simulink model "DAtosInOut_PRBS"  (R2016a)
settings: Solver=ode5  StartTime=0.0  StopTime=t_ejec_anadido  RelTol=1e-3
values from neighbouring files (symbols this model uses):
  D = 1    [Genera_PRBS.m]
  ts = 0.05    [Disena_PRBS.m]    (also in RespuestaStep.m = T)
undefined symbols (not defined in the file or in its folder): sigbuilder_block
libraries: xpcnilib x3, slrtlib x3, simulink x1
Description:
  | Real-Time Controller
  | 
  | This demonstration shows how to build a simple closed-loop real-time controller using
  | Real-Time Windows Target. The output of the controlled plant is connected
  | to the analog input of your data acquisition board. This signal is subtracted from
  | the set point value generated by the signal generator and processed by a PID controller.
  | The output of the controller drives the input of the plant using the analog output
  | of your data acquisition board.
  | 
  | This model is a simplified version of the controller used for the CE152 Magnetic Levitation Model.
  | 
  | How to run this demo:
  | 
  |   1. Open the Analog Input and Analog Output blocks and select your data acquisition board.
  |       If there's no board installed, install it using the Install new board button.
  |   2. Build the model using Tools -> Real-Time Workshop -> Build Model.
  |   3. Connect to the real-time code using Simulation -> Connect to target.
  |   4. Start the real-time execution using Simulation -> Start real-time code.
  | 
  | Note:
  | To run this demo, you must have a data acquisition board plugged into your computer.
settings Model: SimulationMode=external  ExtModeTrigDuration=100000  Creator=Houska  LastModifiedBy=Ainhoa
settings SolverCC: EnableConcurrentExecution=on  AutoInsertRateTranBlk=on
settings DataIOCC: LimitDataPoints=on  MaxDataPoints=P  SaveFormat=Array  SignalLoggingSaveFormat=ModelDataLogs  SignalLoggingName=logsOut
settings OptimizationCC: BlockReduction=off  OptimizeBlockIOStorage=off  BufferReuse=off  GlobalBufferReuse=off  ExpressionFolding=off  ExpressionDepthLimit=2147483647  LocalBlockOutputs=off  InitFltsAndDblsToZero=on  EfficientMapNaN2IntZero=off
settings DebuggingCC: UnderspecifiedInitializationDetection=Classic  MergeDetectMultiDrivingBlocksExec=none  SignalResolutionControl=TryResolveAllWithWarning  FcnCallInpInsideContextMsg=UseLocalSettings  StateNameClashWarn=warning
settings HardwareCC: ProdBitPerPointer=32  ProdLargestAtomicFloat=None  ProdWordSize=32  ProdLongLongMode=on  ProdHWDeviceType=Generic->32-bit x86 compatible
settings ModelReferenceCC: PropagateSignalLabelsOutOfModel=off
settings RTWCC: SystemTargetFile=slrt.tlc  TemplateMakefile=slrt_default_tmf  Description=Simulink Real-Time  RTWCompilerOptimization=on
settings ConfigComp: CovModelRefEnable=Off

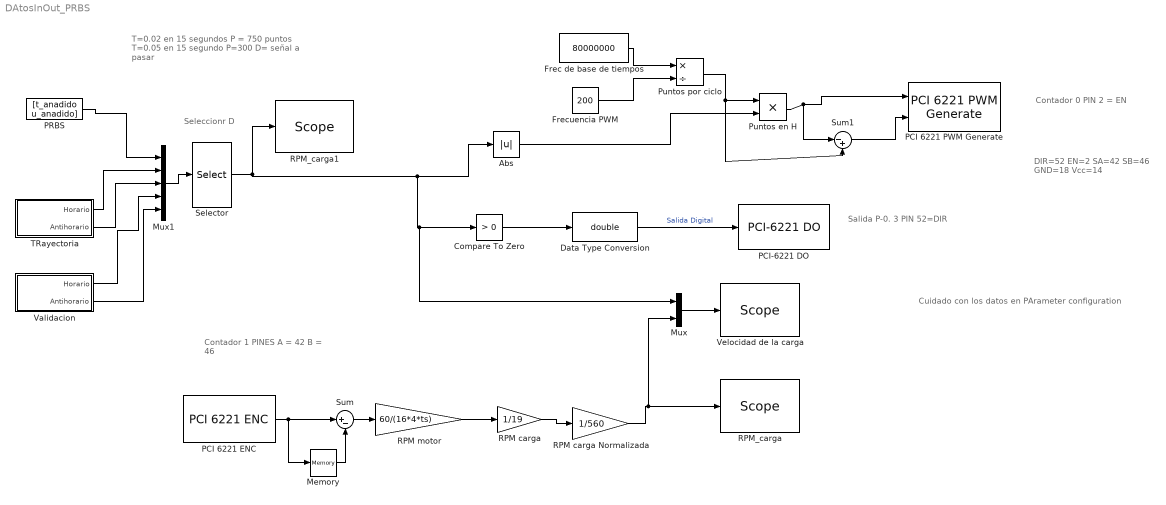
== system DAtosInOut_PRBS ==
  note: Seleccionr D
  note: T=0.02 en 15 segundos P = 750 puntos
      | T=0.05 en 15 segundo P=300
      | D= señal a pasar
  note: Cuidado con los datos en PArameter configuration
  note: DIR=52
      | EN=2
      | SA=42
      | SB=46
      | GND=18
      | Vcc=14
  note: Contador 1
      | PINES
      |  A = 42
      | B = 46
  note: Salida P-0. 3
      | PIN 52=DIR
  note: Contador 0
      | PIN 2 = EN
  Abs : Abs
  Compare To Zero : simulink/Logic and Bit Operations/Compare To Zero  relop=>  OutDataTypeStr=uint8
  Data Type Conversion : DataTypeConversion  OutDataTypeStr=double
  Frec de base de tiempos : Constant  Value=80000000
  Frecuencia PWM : Constant  Value=200
  Memory : Memory
  Mux : Mux  Inputs=2
  Mux1 : Mux  Inputs=5
  "PCI 6221 ENC " : xpcnilib/Incremental Encoder/PCI 6221 ENC   channel=1  countMode=Quadrature Mode x4  initCount=0  reload=off  indexPhase=A low B low  filter=None  sampleTime=ts  slot=-1
  "PCI 6221 PWM Generate " : xpcnilib/Counter/M Series/PCI 6221 PWM Generate   channel=0  initHigh=0  initLow=0  arm=off  disarmlevel=Disarm to LOW  stoplevel=Stop to LOW  sampletime=-1  slot=-1
  PCI-6221 DO : xpcnilib/Digital Output/M Series/PCI-6221 DO  channel=[1]  reset=[1]  initValue=[0]  sampletime=ts  slot=-1
  PRBS : FromWorkspace  VariableName=[t_anadido u_anadido]
  Puntos en H : Product  RndMeth=Zero
  Puntos por ciclo : Product  Inputs=*/
  RPM carga : Gain  Gain=1/19
  RPM carga Normalizada : Gain  Gain=1/560
  RPM motor : Gain  Gain=60/(16*4*ts)
  RPM_carga : slrtlib/Displays and Logging/Scope   scopeno=1  scopetype=File  autostart=on  viewmode=Graphical redraw  formatstr='%15.6f'  grid=on  ylimits=[0,0]  nosamples=P_anadido  noprepostsamples=0  interleave=1  triggermode=FreeRun  triggersignal=1  trigsignalfromport=off  triggerlevel=0.0  triggerslope=Either  triggerscope=1  triggersample=0  filename=salida.dat  mode=Lazy  writesize=512  autorestart=off  dynamicfilemode=off  maxwritefilesize=512*1024^2
  RPM_carga1 : slrtlib/Displays and Logging/Scope   scopeno=2  scopetype=File  autostart=on  viewmode=Graphical redraw  formatstr='%15.6f'  grid=on  ylimits=[0,0]  nosamples=P_anadido  noprepostsamples=0  interleave=1  triggermode=FreeRun  triggersignal=1  trigsignalfromport=off  triggerlevel=0.0  triggerslope=Either  triggerscope=1  triggersample=0  filename=entrada.dat  mode=Lazy  writesize=512  autorestart=off  dynamicfilemode=off  maxwritefilesize=512*1024^2
  Selector : Selector  InputPortWidth=5  IndexOptions=Index vector (dialog)  Indices=[D]  OutputSizes=1
  Sum : Sum  Inputs=|+-
  Sum1 : Sum  Inputs=|-+
  TRayectoria : Subsystem  Tag=STV Subsys  LoadFcn=sigbuilder_block('load');  StartFcn=sigbuilder_block('start');  StopFcn=sigbuilder_block('stop');  ClipboardFcn=sigbuilder_block('clipboard');  mask(Sigbuilder block){}
      mask help: Simulink:masks:SigbuilderBlock_MD
      mask init:
      | if ~strcmp(get_param(bdroot(gcbh),'SimulationStatus'),'stopped') tuvar = sigbuilder_block('maskInit'); end
      settings: CopyFcn=sigbuilder_block('copy');  DeleteFcn=sigbuilder_block('delete');  ModelCloseFcn=sigbuilder_block('modelClose');  PreSaveFcn=sigbuilder_block('preSave');  PauseFcn=sigbuilder_block('pause');  ContinueFcn=sigbuilder_block('continue');  NameChangeFcn=sigbuilder_block('namechange');  OpenFcn=sigbuilder_block('open',[6 6 1188 718.5 ]);  CloseFcn=sigbuilder_block('close');
      mask Display: plot(0, 0, 100, 100,[2, 2, 32, 32, 2], [68, 8, 8, 68, 68],[32, 2], [38, 38], [32, 19, 2],[53, 60, 44], [32, 17, 17, 2],[16, 16, 31, 31]);txt = getActiveGroup(gcbh);text(2, 100, txt,'verticalAlignment', 'top');
  Validacion : Subsystem  Tag=STV Subsys  LoadFcn=sigbuilder_block('load');  StartFcn=sigbuilder_block('start');  StopFcn=sigbuilder_block('stop');  ClipboardFcn=sigbuilder_block('clipboard');  mask(Sigbuilder block){}
      mask help: Simulink:masks:SigbuilderBlock_MD
      mask init:
      | if ~strcmp(get_param(bdroot(gcbh),'SimulationStatus'),'stopped') tuvar = sigbuilder_block('maskInit'); end
      settings: CopyFcn=sigbuilder_block('copy');  DeleteFcn=sigbuilder_block('delete');  ModelCloseFcn=sigbuilder_block('modelClose');  PreSaveFcn=sigbuilder_block('preSave');  PauseFcn=sigbuilder_block('pause');  ContinueFcn=sigbuilder_block('continue');  NameChangeFcn=sigbuilder_block('namechange');  OpenFcn=sigbuilder_block('open',[43.5 -15.75 1188 714 ]);  CloseFcn=sigbuilder_block('close');
      mask Display: plot(0, 0, 100, 100,[2, 2, 32, 32, 2], [68, 8, 8, 68, 68],[32, 2], [38, 38], [32, 19, 2],[53, 60, 44], [32, 17, 17, 2],[16, 16, 31, 31]);txt = getActiveGroup(gcbh);text(2, 100, txt,'verticalAlignment', 'top');
  Velocidad de la carga : slrtlib/Displays and Logging/Scope   scopeno=3  scopetype=Host  autostart=on  viewmode=Graphical redraw  formatstr='%15.6f'  grid=on  ylimits=[0,0]  nosamples=P_anadido  noprepostsamples=1  interleave=1  triggermode=FreeRun  triggersignal=1  trigsignalfromport=off  triggerlevel=0.0  triggerslope=Either  triggerscope=1  triggersample=0  filename=data.dat  mode=Lazy  writesize=512  autorestart=off  dynamicfilemode=off  maxwritefilesize=512*1024^2
  wires:
  "PCI 6221 ENC "/1 -> Memory/1, Sum/1
  Memory/1 -> Sum/2
  Sum/1 -> RPM motor/1
  RPM carga/1 -> RPM carga Normalizada/1
  RPM motor/1 -> RPM carga/1
  Sum1/1 -> "PCI 6221 PWM Generate "/2
  Frec de base de tiempos/1 -> Puntos por ciclo/1
  Frecuencia PWM/1 -> Puntos por ciclo/2
  Puntos por ciclo/1 -> Puntos en H/1, Sum1/2
  Puntos en H/1 -> "PCI 6221 PWM Generate "/1, Sum1/1
  Data Type Conversion/1 -> PCI-6221 DO/1  "Salida Digital"
  Abs/1 -> Puntos en H/2
  Compare To Zero/1 -> Data Type Conversion/1
  RPM carga Normalizada/1 -> Mux/2, RPM_carga/1
  Mux/1 -> Velocidad de la carga/1
  Selector/1 -> RPM_carga1/1, Mux/1, Compare To Zero/1, Abs/1
  PRBS/1 -> Mux1/1
  Mux1/1 -> Selector/1
  TRayectoria/1(Horario) -> Mux1/2
  TRayectoria/2(Antihorario) -> Mux1/3
  Validacion/1(Horario) -> Mux1/4
  Validacion/2(Antihorario) -> Mux1/5

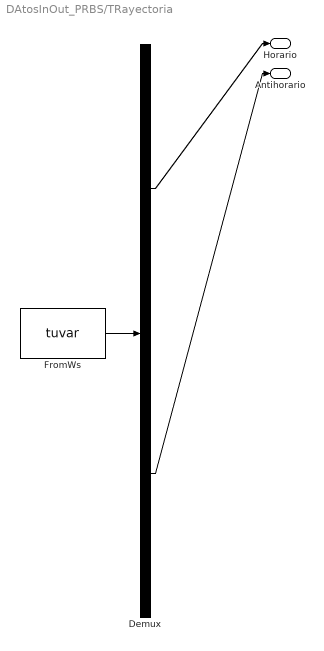
== system DAtosInOut_PRBS/TRayectoria ==
  Demux : Demux  Tag=STV Demux  Outputs=2
  FromWs : FromWorkspace  Tag=STV FromWs  VariableName=tuvar  SampleTime=0
      SigBuilderData=|
      | common.afterFinalStr = 'Extrapolate'
      | common.sampleTime = 0
      | dataSet.timeRange = [0 15]
      | dataSet.name = 'Trayectoria'
      | sbobj.Groups.Name = 'Trayectoria'
      | sbobj.Groups.Signals(1).Name = 'Horario'
      | sbobj.Groups.Signals(1).XData = [0 1 2.02 2.34 2.34 3 4 4 4.64 5.32 5.32 6 7 8 9 10 11.94 11.94 12.28 12.3 12.7 12.7 15]
      | sbobj.Groups.Signals(1).YData = [0.2 0.4 0.2 0.2 0.4 0.4 0.2 0.3 0.3 0.5 0.4 0.4 0.3 0.4 0.2 0.2 0.5 0.2 0.2 0.3 0.3 0.4 0.2]
      | sbobj.Groups.Signals(2).Name = 'Antihorario'
      | sbobj.Groups.Signals(2).XData = [0 1 2 2.38 2.38 3 3 4 4 4.62 5.3 5.3 6 6 7 8 9.02 10 12 12 12.4 12.4 12.78 12.78 15]
      | sbobj.Groups.Signals(2).YData = [-0.2 -0.6 -0.2 -0.2 -0.8 -0.8 -0.6 -0.2 -0.8 -0.8 -0.6 -0.4 -0.4 -0.6 -0.8 -0.4 -0.2 -0.2 -0.7 -0.2 -0.2 -0.5 -0.5 -0.3 -0.2]
      | sbobj.Groups.TimeRange = [0 15]
  Horario : Outport  Tag=STV Outport
  Antihorario : Outport  Tag=STV Outport  Port=2
  wires:
  FromWs/1 -> Demux/1
  Demux/1 -> Horario/1
  Demux/2 -> Antihorario/1

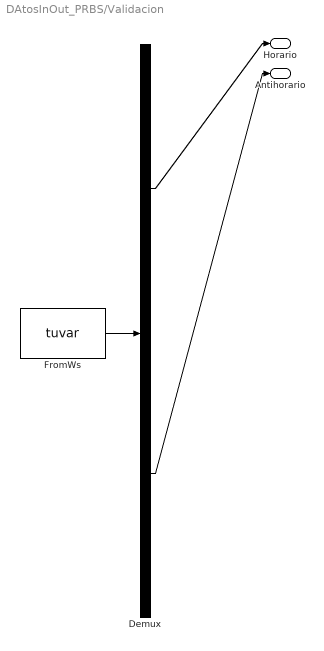
== system DAtosInOut_PRBS/Validacion ==
  Demux : Demux  Tag=STV Demux  Outputs=2
  FromWs : FromWorkspace  Tag=STV FromWs  VariableName=tuvar  SampleTime=0
      SigBuilderData=|
      | common.afterFinalStr = 'Extrapolate'
      | common.sampleTime = 0
      | dataSet.timeRange = [0 15]
      | dataSet.name = 'Validacion'
      | sbobj.Groups.Name = 'Validacion'
      | sbobj.Groups.Signals(1).Name = 'Horario'
      | sbobj.Groups.Signals(1).XData = [0 0.8 1.5 1.7 2.34 3 3 3.6 3.6 3.9 4.3 5 6.1 6.9 6.9 7.4 7.4 7.9 7.9 8.4 8.4 10 11.94 11.94 12.28 12.3 12.7 15]
      | sbobj.Groups.Signals(1).YData = [0.2 0.4 0.4 0.3 0.4 0.4 0.2 0.2 0.4 0.4 0.3 0.3 0.4 0.4 0.2 0.2 0.4 0.4 0.2 0.2 0.4 0.2 0.4 0.2 0.2 0.4 0.4 0.2]
      | sbobj.Groups.Signals(2).Name = 'Antihorario'
      | sbobj.Groups.Signals(2).XData = [0 0.5 1.6 1.6 2.38 3 3 3.6 3.6 3.9 3.9 4.3 4.3 6 7 7 7.9 7.9 10 12 12 12.4 12.4 12.78 12.78 15]
      | sbobj.Groups.Signals(2).YData = [-0.2 -0.6 -0.8 -0.4 -0.8 -0.8 -0.2 -0.2 -0.4 -0.4 -0.6 -0.6 -0.8 -0.4 -0.4 -0.2 -0.2 -0.8 -0.2 -0.8 -0.2 -0.2 -0.8 -0.8 -0.4 -0.2]
      | sbobj.Groups.TimeRange = [0 15]
  Horario : Outport  Tag=STV Outport
  Antihorario : Outport  Tag=STV Outport  Port=2
  wires:
  FromWs/1 -> Demux/1
  Demux/1 -> Horario/1
  Demux/2 -> Antihorario/1
